simulink model "flightControlSystem"  (R2024a)
settings: Solver=ode3  StartTime=0  StopTime=TFinal  FixedStep=Ts  RelTol=1e-3  EnableMultiTasking=on
undefined symbols (not defined in the file): codertarget, Controller, DiscIntNeverNeededParam, Discrete, Estimator, g, gray, init, orient_ref, pos_ref, Sensors, Time, Ts, var_acc_angle_N, var_bias_gyr_N, var_gyro_p_N, Vehicle
libraries: simulink x55, slpidlib x4, ctrlSharedLib x4, sharedtransform x3, parrotlib x1
(part 3 of 3)

== system flightControlSystem/Control System/State Estimator/XY Position Estimator/EstimatorVelocity/xy velocity w//o angular velocity compensation ==
  note: Optical flow raw readings are converted to velocity in m/s based on the estimated altitude
  optical_flow : Inport
  z_estimate : Inport  Port=2
  " " : Product  Inputs=**
  Compare To Constant : simulink/Logic and Bit Operations/Compare To Constant  relop=<  const=200*4  OutDataTypeStr=boolean
  Counter Free-Running : simulink/Sources/Counter Free-Running  NumBits=32  tsamp=-1
  Gain : Gain  Gain=-1
  Select dxy : Selector  InputPortWidth=3  IndexOptions=Index vector (dialog)  Indices=[1 2]  OutputSizes=1
  Switch : Switch  Criteria=u2 > Threshold  SaturateOnIntegerOverflow=off  InputSameDT=off
  opticalFlowErrorCorrect : Gain  Gain=1.15
  optical_flow_dx_dy : Outport
  wires:
  Select dxy/1 -> optical_flow_dx_dy/1  "optical_flow_dx_dy"
  " "/1 -> opticalFlowErrorCorrect/1
  opticalFlowErrorCorrect/1 -> Switch/3
  Gain/1 -> " "/2
  Switch/1 -> Select dxy/1
  Counter Free-Running/1 -> Compare To Constant/1
  Compare To Constant/1 -> Switch/2
  optical_flow/1 -> " "/1, Switch/1
  z_estimate/1 -> Gain/1

== matlab function flightControlSystem/Image Processing System/MATLAB Function ==
  data: boolVector input; result output
function result = evaluateBooleanVector(boolVector)
    % Check if input is a logical vector
    if ~islogical(boolVector)
        error('Input must be a logical vector');
    end

    % Count the number of true and false values
    numTrue = sum(boolVector);
    numFalse = length(boolVector) - numTrue;

    % Return 1 if number of true values is greater, otherwise return 0
    if numTrue > numFalse
        result = 1;
    else
        result = 0;
    end
end

== matlab function flightControlSystem/Control System/Controller/Position Controller/Position error transformation (Earth to Body frame) ==
  data: yaw input; xy_err_earth input; xy_err_body output
function xy_err_body = fcn(yaw,xy_err_earth)

transformation = [cos(yaw), sin(yaw); -sin(yaw),  cos(yaw)];
xy_err_body = transformation * xy_err_earth;


end

== stateflow chart flightControlSystem/Control System/Path Planning/Chart ==
  state Landing [group]
    state Search_landing
      during:
      vel=0.0005
      xout=xout+pcos(vel,yaw);
      yout=yout+psin(vel,yaw);
      off_dis=off_dis+1
    state No_landing
      during:
      vel=-0.0005
      xout=xout+pcos(vel,yaw);
      yout=yout+psin(vel,yaw);
      off_dis=off_dis-1;
    Search_landing -> (junction 159) : [r32==0]
    (junction 159) -> No_landing [order 2] : [r22==0&&r12==0]
  state Forward
    during:
    vel=0.0005;
    xout=xout+pcos(vel,yaw);
    yout=yout+psin(vel,yaw);
    zout=-0.5;
    off_dis=0;
  state Startup
    entry:
    zout=0;
    yout=0;
    xout=0;
    yaw=0;
    vel=0;
    flg=0;
  state Hover
    during:
    xout=xout;
    yout=yout;
    zout=-0.7;
  state Rise
    during:
    zout=-0.7;
  state Fall
    during:
    zout=-0.001;
  state End
    exit:
  state Turning [group]
    state R_turn
      during:
      vel=0;
      yaw=yaw+(22/7)/1000;
    state L_turn
      during:
      vel=0;
      yaw=yaw-(22/7)/1000;
    R_turn -> (junction 174) [order 2] : [r12==1]
    L_turn -> (junction 174) [order 1] : [r12==1]
    (junction 172) -> R_turn [order 1] : [(r13==1||r33==1)&&(r11==0&&r31==0)]
    (junction 172) -> L_turn [order 2] : [(r11==1||r31==1)&&(r13==0&&r33==0)]
  state Stabilize [group]
    state L_align
      during:
      vel=0.00015;
      xout=xout+psin(vel,yaw);
      yout=yout-pcos(vel,yaw);
      counter=counter-1;
    state R_align
      during:
      vel=-0.0002;
      xout=xout+psin(vel,yaw);
      yout=yout-pcos(vel,yaw);
      counter=counter-1;
    (junction 165) -> R_align [order 1] : [(r23==1)&&(r33==1)&&(r13==0)&&(r31==0)&&flg==0]{counter=10;}
    (junction 165) -> L_align [order 2] : [(r21==1)&&(r31==1)&&(r11==0)&&(r33==0)&&flg==0]{counter=10;}
    (junction 167) -> (junction 165)
    L_align -> (junction 167) : [((r11==0)&&(r31==0))||(counter<=0)]
    R_align -> (junction 167) : [((r13==0)&&(r33==0))||(counter<=0)]
  state Stop_crash
    during:
    zout=0.7
  state Forward2
    during:
    xout=xout+0.0005;
    yout=0;
    zout=-0.5;
  state Checker
    during:
    xout=xout;
    yout=yout+0.0005;
  state Landing2
    during:
    zout=0.7
  state Right_
    during:
    xout=xout;
    yaw=yaw+0.0005
  state Backward
    during:
    yout=yout+0.0005;
    zout=-0.7;
  (junction 159) -> Fall [order 1] : [(r22==1&&r12==1)||(r22==1&&r32==0)]
  Hover -> Search_landing [order 2] : [(r12==0)&& ...
      | (r11==0)&&(r21==0)&& ...
      | (r13==0)&&(r23==0)&& ...
      | (flg==0)]{flg=1;off_dis=0;}
  No_landing -> Hover : [(r22==1)&&(off_dis<=0)]
  (default) -> Startup
  Hover -> Forward [order 1] : [r12==1&&r22==1]
  Forward -> Fall [order 2] : [r22==0]
  Startup -> Rise : [r11==1 && r12==1&&r13==1&& ...
      | r21==1&&r22==1&&r23==1&& ...
      | r31==1&&r32==1&&r33==1]
  Rise -> Hover : [r11==0&&r13==0&& ...
      | r31==0&&r33==0&& ...
      | r22==1]
  Fall -> End : after(2,sec)
  Forward -> Hover [order 1] : [r12==0]
  L_turn -> Fall [order 2] : [r22==0]
  R_turn -> Fall [order 1] : [r22==0]
  (junction 165) -> Hover [order 4]
  Hover -> (junction 165) [order 3] : [r12==0]
  (junction 174) -> Hover : {flg=0;}
  (junction 165) -> (junction 172) [order 3] : [r12==0]
  Forward2 -> Checker [order 2] : [r12==0&&r22==0]
  Checker -> Stop_crash [order 2] : [after(3,sec) && r12==0 && r22==0]
  Forward2 -> Right_ [order 1] : [r13==1]
  Checker -> Landing2 [order 1] : [after(3.05,sec) && r12==1 || r22==1]
  Right_ -> Backward : [r12==1 &&r13==0&& r23==1 && r22==1]
  Backward -> Checker : [r12==0&&r22==0 ]
  data: a function_input; rad function_input; x function_output; a function_input; rad function_input; y function_output; eZ input; eY input; eX input; r11 input; xout output; yout output; zout output; yaw output; r12 input; r22 input; r13 input; r21 input; r23 input; r31 input; r32 input; r33 input; flg local; off_dis local; counter local; vel local
  function x = psin(a,rad):
    | function x = psin(a,rad)
    |     x = double(a*sin(rad));
    | end
  function y = pcos(a,rad):
    | function y = pcos(a,rad)
    |     y = double(a*cos(rad));
    | end

== matlab function flightControlSystem/Image Processing System/MATLAB Function1 ==
  data: boolVector input; result output
function result = evaluateBooleanVector(boolVector)
    % Check if input is a logical vector
    if ~islogical(boolVector)
        error('Input must be a logical vector');
    end

    % Count the number of true and false values
    numTrue = sum(boolVector);
    numFalse = length(boolVector) - numTrue;

    % Return 1 if number of true values is greater, otherwise return 0
    if numTrue > numFalse
        result = 1;
    else
        result = 0;
    end
end

== matlab function flightControlSystem/Image Processing System/MATLAB Function2 ==
  data: boolVector input; result output
function result = evaluateBooleanVector(boolVector)
    % Check if input is a logical vector
    if ~islogical(boolVector)
        error('Input must be a logical vector');
    end

    % Count the number of true and false values
    numTrue = sum(boolVector);
    numFalse = length(boolVector) - numTrue;

    % Return 1 if number of true values is greater, otherwise return 0
    if numTrue > numFalse
        result = 1;
    else
        result = 0;
    end
end

== matlab function flightControlSystem/Image Processing System/MATLAB Function3 ==
  data: boolVector input; result output
function result = evaluateBooleanVector(boolVector)
    % Check if input is a logical vector
    if ~islogical(boolVector)
        error('Input must be a logical vector');
    end

    % Count the number of true and false values
    numTrue = sum(boolVector);
    numFalse = length(boolVector) - numTrue;

    % Return 1 if number of true values is greater, otherwise return 0
    if numTrue > numFalse
        result = 1;
    else
        result = 0;
    end
end

== matlab function flightControlSystem/Image Processing System/MATLAB Function4 ==
  data: boolVector input; result output
function result = evaluateBooleanVector(boolVector)
    % Check if input is a logical vector
    if ~islogical(boolVector)
        error('Input must be a logical vector');
    end

    % Count the number of true and false values
    numTrue = sum(boolVector);
    numFalse = length(boolVector) - numTrue;

    % Return 1 if number of true values is greater, otherwise return 0
    if numTrue > numFalse
        result = 1;
    else
        result = 0;
    end
end

== matlab function flightControlSystem/Image Processing System/MATLAB Function5 ==
  data: boolVector input; result output
function result = evaluateBooleanVector(boolVector)
    % Check if input is a logical vector
    if ~islogical(boolVector)
        error('Input must be a logical vector');
    end

    % Count the number of true and false values
    numTrue = sum(boolVector);
    numFalse = length(boolVector) - numTrue;

    % Return 1 if number of true values is greater, otherwise return 0
    if numTrue > numFalse
        result = 1;
    else
        result = 0;
    end
end

== matlab function flightControlSystem/Image Processing System/MATLAB Function6 ==
  data: boolVector input; result output
function result = evaluateBooleanVector(boolVector)
    % Check if input is a logical vector
    if ~islogical(boolVector)
        error('Input must be a logical vector');
    end

    % Count the number of true and false values
    numTrue = sum(boolVector);
    numFalse = length(boolVector) - numTrue;

    % Return 1 if number of true values is greater, otherwise return 0
    if numTrue > numFalse
        result = 1;
    else
        result = 0;
    end
end

== matlab function flightControlSystem/Image Processing System/MATLAB Function7 ==
  data: boolVector input; result output
function result = evaluateBooleanVector(boolVector)
    % Check if input is a logical vector
    if ~islogical(boolVector)
        error('Input must be a logical vector');
    end

    % Count the number of true and false values
    numTrue = sum(boolVector);
    numFalse = length(boolVector) - numTrue;

    % Return 1 if number of true values is greater, otherwise return 0
    if numTrue > numFalse
        result = 1;
    else
        result = 0;
    end
end

== matlab function flightControlSystem/Image Processing System/MATLAB Function8 ==
  data: boolVector input; result output
function result = evaluateBooleanVector(boolVector)
    % Check if input is a logical vector
    if ~islogical(boolVector)
        error('Input must be a logical vector');
    end

    % Count the number of true and false values
    numTrue = sum(boolVector);
    numFalse = length(boolVector) - numTrue;

    % Return 1 if number of true values is greater, otherwise return 0
    if numTrue > numFalse
        result = 1;
    else
        result = 0;
    end
end
